simulink model "fourinputslq_and_yaw_rate_control_sim"  (R2015a)
settings: Solver=ode3  SolverMode=SingleTasking  StartTime=0.0  StopTime=10.0  FixedStep=ts  RelTol=1e-3
values from neighbouring files (symbols this model uses):
  Cs = [1 0 0 0 0 0; 0 1 0 0 0 0; 0 0 1 0 0 0;  0 0 0 1 0 0;0 0 0 0 1 0]    [fourinputslq_and_yaw_rate_control.m]    (also in matlab.mat = [1 0 0 0 0 0 1 0 0 0 0 0 ... (30 elements, 5x6)])
  Kd = [-1.6913845986 -1.69122939247 1.69176062912 1.69191583525 -1.69161510275 1.69114487429 1.69153012497 -1.69200035344 -9089.91497099 9076.05839329 -9089.91497099 9076.05839329 ... (20 elements, 4x5)]    [matlab.mat]
settings Model: Creator=Jaby  LastModifiedBy=Jaby
settings OptimizationCC: BlockReduction=off  BooleanDataType=off
settings DebuggingCC: SaveWithParameterizedLinksMsg=none  UnderspecifiedInitializationDetection=Classic  MergeDetectMultiDrivingBlocksExec=none  SignalResolutionControl=TryResolveAllWithWarning
settings HardwareCC: TargetUnknown=on

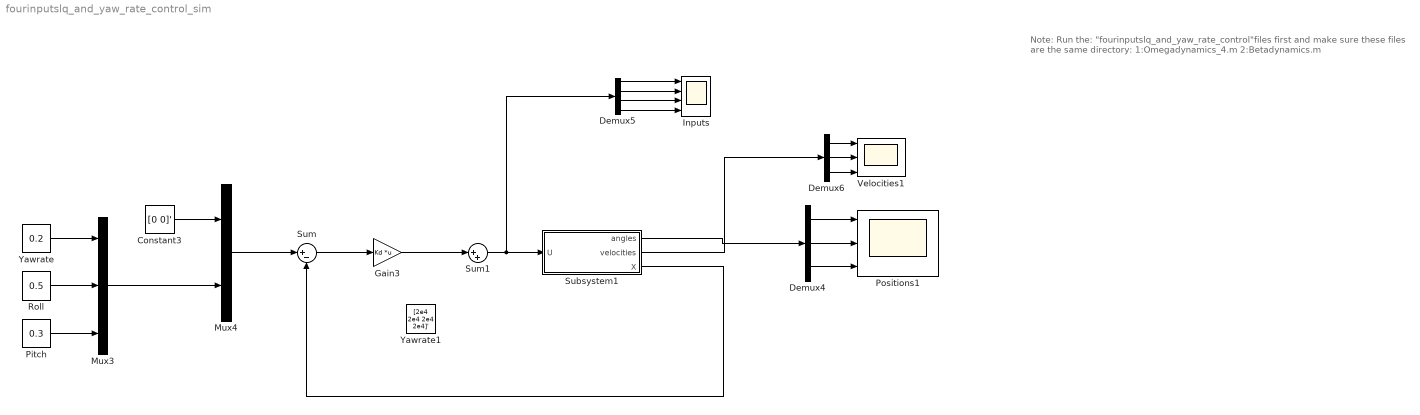
== system fourinputslq_and_yaw_rate_control_sim ==
  note: Note:
      | Run the: "fourinputslq_and_yaw_rate_control"files first and make sure these files are the same directory:
      | 1:Omegadynamics_4.m
      | 2:Betadynamics.m
  Constant3 : Constant  Value=[0 0]'  VectorParams1D=off
  Demux4 : Demux  Outputs=3
  Demux5 : Demux
  Demux6 : Demux  Outputs=3
  Gain3 : Gain  Gain=Kd  Multiplication=Matrix(K*u)
  Inputs : Scope  NumInputPorts=4
      settings: TimeRange=20  YMin=0.00274~-3.07e-14~8.3e-31~-5  YMax=0.00278~-3.025e-14~8.43e-31~5  SaveName=ScopeData4
  Mux3 : Mux  Inputs=3
  Mux4 : Mux  Inputs=2
  Pitch : Constant  Value=0.3
  Positions1 : Scope  NumInputPorts=3
      settings: TimeRange=10  YMin=0.19775~0.149~1.5  YMax=0.20025~0.155~4.75  SaveName=ScopeData5
  Roll : Constant  Value=0.5
  Subsystem1 : Subsystem
  Sum : Sum  Inputs=|+-
  Sum1 : Sum  Inputs=|++
  Velocities1 : Scope  NumInputPorts=3
      settings: TimeRange=10  YMin=-0.083~0.096~0.475  YMax=-0.076~0.1015~0.525  SaveName=ScopeData9
  Yawrate : Constant  Value=0.2
  Yawrate1 : Constant  Value=[2e4 2e4 2e4 2e4]'  VectorParams1D=off
  wires:
  Demux4/2 -> Positions1/2
  Demux4/3 -> Positions1/3
  Demux4/1 -> Positions1/1
  Demux6/2 -> Velocities1/2
  Demux6/3 -> Velocities1/3
  Demux6/1 -> Velocities1/1
  Subsystem1/1(angles) -> Demux4/1
  Subsystem1/2(velocities) -> Demux6/1
  Roll/1 -> Mux3/2
  Pitch/1 -> Mux3/3
  Mux4/1 -> Sum/1
  Mux3/1 -> Mux4/2
  Constant3/1 -> Mux4/1
  Sum/1 -> Gain3/1
  Yawrate/1 -> Mux3/1
  Subsystem1/3(X) -> Sum/2
  Demux5/1 -> Inputs/1
  Demux5/2 -> Inputs/2
  Demux5/3 -> Inputs/3
  Demux5/4 -> Inputs/4
  Gain3/1 -> Sum1/1
  Sum1/1 -> Subsystem1/1(U), Demux5/1

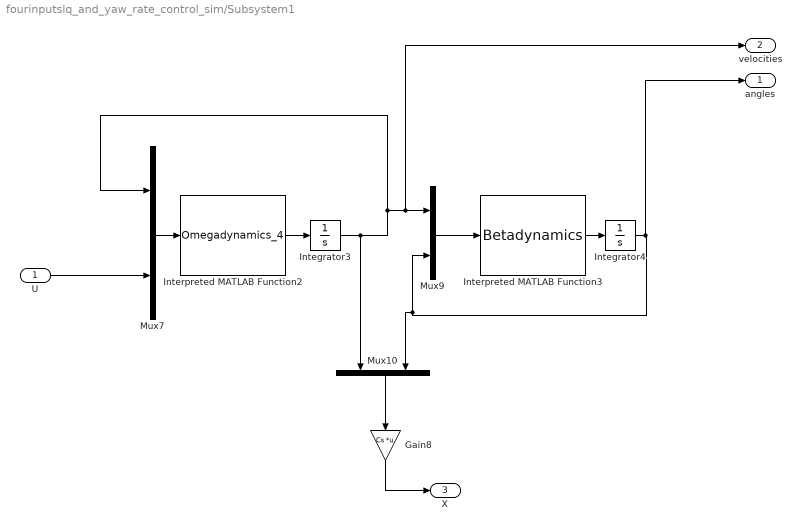
== system fourinputslq_and_yaw_rate_control_sim/Subsystem1 ==
  U : Inport
  Gain8 : Gain  Gain=Cs  Multiplication=Matrix(K*u)
  Integrator3 : Integrator  InitialCondition=[0 0 0]'
  Integrator4 : Integrator  InitialCondition=[0 0 0]'
  Interpreted MATLAB Function2 : MATLABFcn  MATLABFcn=Omegadynamics_4  Output1D=off
  Interpreted MATLAB Function3 : MATLABFcn  MATLABFcn=Betadynamics  Output1D=off
  Mux10 : Mux  Inputs=2
  Mux7 : Mux  Inputs=2
  Mux9 : Mux  Inputs=2
  angles : Outport
  velocities : Outport  Port=2
  X : Outport  Port=3
  wires:
  Gain8/1 -> X/1
  U/1 -> Mux7/2
  Integrator4/1 -> Mux10/2, Mux9/2, angles/1
  Mux9/1 -> Interpreted MATLAB Function3/1
  Mux10/1 -> Gain8/1
  Interpreted MATLAB Function3/1 -> Integrator4/1
  Interpreted MATLAB Function2/1 -> Integrator3/1
  Mux7/1 -> Interpreted MATLAB Function2/1
  Integrator3/1 -> Mux10/1, Mux9/1, velocities/1, Mux7/1
